simulink model "automata_learning"  (R2022a)
settings: Solver=FixedStepAuto  StartTime=0.0  StopTime=10.0  FixedStep=0.05  RelTol=1e-3
settings Model: Creator=diego  LastModifiedBy=diego

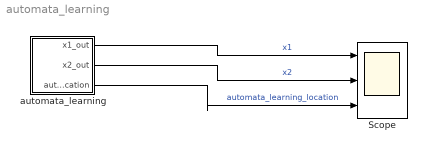
== system automata_learning ==
  Scope : Scope  NumInputPorts=3
  automata_learning : Stateflow chart  TreatAsAtomicUnit=on
  wires:
  automata_learning/1(x1_out) -> Scope/1  "x1"
  automata_learning/2(x2_out) -> Scope/2  "x2"
  automata_learning/3(automata_learning_location) -> Scope/3  "automata_learning_location"

== stateflow chart automata_learning/automata_learning ==
  settings: updateMethod=CONTINUOUS
  state loc1
    du:
    x1_dot = 0.002086562738824682 * x2 - 0.06258858929709277 * x1 + 1.0731875028614013;
    x2_dot = 0.7014102662978985 * x1 + 0.004290363107898543 * x2 + 0.3763837828655596;
    x1_out=x1;
    x2_out=x2;
    automata_learning_location =1;
  state loc2
    du:
    x1_dot = 0.10104580940196684 * x1 - 0.044842719787084206 * x2 - 0.4112039586834726;
    x2_dot = 0.027354503509286587 * x1 - 0.0006732579461932175 * x2 + 0.8892702702814859;
    x1_out=x1;
    x2_out=x2;
    automata_learning_location =2;
  loc1 -> loc2 : [0.0000005511 * x2 - 0.2482 * x1 + 1.0 < 0.0]
  (default) -> loc1 : {x1 = 0.0;
      | x2 = 0.0;}
  loc2 -> loc1 : [43.09132960916031 * x1 + 0.021145646542095164 * x2 + 1.0 < 0.0 && -75.02048562094569 * x1 - 0.1991395009226835 * x2 + 1.0 > 0.0]
  data: x1_out output; x1 local; x2_out output; x2 local; automata_learning_location output
  data x1 settings: updateMethod=SF_CONTINUOUS_TIME_DATA
  data x2 settings: updateMethod=SF_CONTINUOUS_TIME_DATA
